simulink model "trial"  (R2021a)
settings: Solver=VariableStepAuto  StartTime=0.0  StopTime=10.0  RelTol=1e-3
settings Model: Creator=Saniya  LastModifiedBy=Saniya

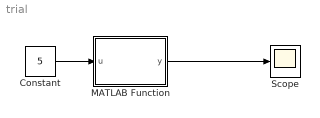
== system trial ==
  Constant : Constant  Value=5
  MATLAB Function : MATLAB Function  TreatAsAtomicUnit=on
  Scope : Scope
  wires:
  MATLAB Function/1(y) -> Scope/1
  Constant/1 -> MATLAB Function/1(u)

== matlab function trial/MATLAB Function ==
  data: u input; y output
function y = fcn(u)
y = zeros(1, 'double');
coder.extrinsic('sumodd_mex');
y=sumodd_mex(u);
end
